simulink model "snowpack_scheduler"  (R2014a)
settings: Solver=FixedStepDiscrete  StartTime=0.0  StopTime=10.0  FixedStep=0.01  RelTol=1e-3
settings Model: Creator=The MathWorks Inc.  LastModifiedBy=feisele
settings OptimizationCC: ExpressionDepthLimit=2147483647
settings DebuggingCC: UnderspecifiedInitializationDetection=Classic  FcnCallInpInsideContextMsg=UseLocalSettings  StateNameClashWarn=warning
settings SFSimCC: SimParseCustomCode=off
settings GRTTargetCC: CombineOutputUpdateFcns=off  GRTInterface=on

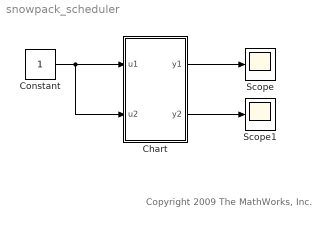
== system snowpack_scheduler ==
  note: Copyright 2009 The MathWorks, Inc.
  Chart : Stateflow chart  TreatAsAtomicUnit=on
  Constant : Constant
  Scope : Scope
      settings: YMin=0  YMax=350
  Scope1 : Scope
      settings: YMin=0  YMax=350
  wires:
  Constant/1 -> Chart/1(u1), Chart/2(u2)
  Chart/1(y1) -> Scope/1
  Chart/2(y2) -> Scope1/1

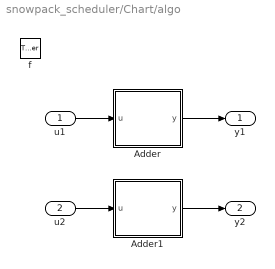
== system snowpack_scheduler/Chart/algo ==
  u1 : Inport
  u2 : Inport  Port=2
  f : TriggerPort  TriggerType=function-call
      settings: CopyFcn=Stateflow.SLINSF.SimulinkMan.removeBlockPreDeleteFcn  PreDeleteFcn=Stateflow.SLINSF.SimulinkMan.unsafePredeleteFcn
  Adder : Subsystem
  Adder1 : Subsystem
  y1 : Outport
  y2 : Outport  Port=2
  wires:
  u1/1 -> Adder/1(u)
  Adder/1(y) -> y1/1
  u2/1 -> Adder1/1(u)
  Adder1/1(y) -> y2/1

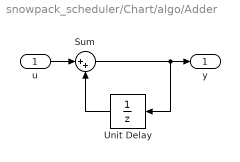
== system snowpack_scheduler/Chart/algo/Adder ==
  u : Inport
  Sum : Sum  Inputs=|++
  Unit Delay : UnitDelay  SampleTime=-1
  y : Outport
  wires:
  Sum/1 -> Unit Delay/1, y/1
  Unit Delay/1 -> Sum/2
  u/1 -> Sum/1

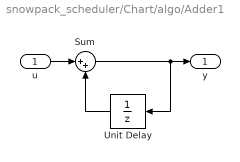
== system snowpack_scheduler/Chart/algo/Adder1 ==
  u : Inport
  Sum : Sum  Inputs=|++
  Unit Delay : UnitDelay  SampleTime=-1
  y : Outport
  wires:
  u/1 -> Sum/1
  Unit Delay/1 -> Sum/2
  Sum/1 -> y/1, Unit Delay/1

== stateflow chart snowpack_scheduler/Chart ==
  state FAST
    on every(2,tick): [y1,y2] = algo(u1,u2);
  state SLOW
    on every(5,tick): [y1,y2] = algo(u1,u2);
  state [y1,y2] = algo(u1,u2) [function]
  (default) -> FAST
  FAST -> SLOW : after(50,tick)
  SLOW -> FAST : after(75,tick)
  data: u1 function_input; u2 function_input; y1 function_output; y2 function_output; u1 input double; u2 input double; y1 output double; y2 output double
